simulink model "MS_QD2_QBPlat_R2021a"  (R2021a)
settings: Solver=ode2  StartTime=0.0  StopTime=inf  FixedStep=0.001  RelTol=1e-3  EnableMultiTasking=on
undefined symbols (not defined in the file): Host, localhost, qc_get_step_size
libraries: quarc_library x71, simulink x10, simulink_extras x2
(part 2 of 2)

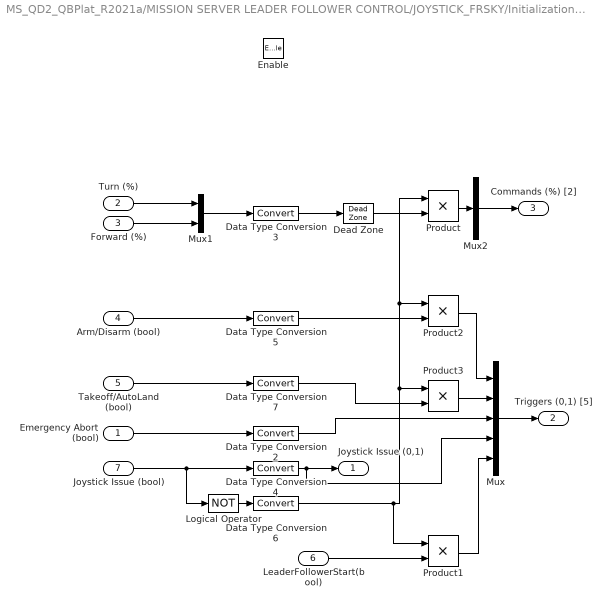
== system MS_QD2_QBPlat_R2021a/MISSION SERVER LEADER FOLLOWER CONTROL/JOYSTICK_FRSKY/Initialization and Conditioning ==
  Emergency Abort (bool) : Inport
  Turn (%) : Inport  Port=2
  Forward (%) : Inport  Port=3
  Arm/Disarm (bool) : Inport  Port=4
  Takeoff/AutoLand (bool) : Inport  Port=5
  LeaderFollowerStart(bool) : Inport  Port=6
  Joystick Issue (bool) : Inport  Port=7
  Enable : EnablePort  StatesWhenEnabling=reset
  Data Type Conversion{2..7} (6 alike) : DataTypeConversion
  Dead Zone : DeadZone  LowerValue=-0.01  UpperValue=0.01  SaturateOnIntegerOverflow=on
  Logical Operator : Logic  Operator=NOT  AllPortsSameDT=off  OutDataTypeStr=boolean
  Mux : Mux  Inputs=5
  Mux1 : Mux  Inputs=2
  Mux2 : Mux  Inputs=1
  Product{,1..3} (4 alike) : Product
  Joystick Issue (0,1) : Outport  InitialOutput=0  VectorParamsAs1DForOutWhenUnconnected=off
  Triggers (0,1) [5] : Outport  Port=2  InitialOutput=0  VectorParamsAs1DForOutWhenUnconnected=off
  Commands (%) [2] : Outport  Port=3  InitialOutput=0  VectorParamsAs1DForOutWhenUnconnected=off
  wires:
  Joystick Issue (bool)/1 -> Data Type Conversion4/1, Logical Operator/1
  Mux1/1 -> Data Type Conversion3/1
  Turn (%)/1 -> Mux1/1
  Forward (%)/1 -> Mux1/2
  Data Type Conversion4/1 -> Joystick Issue (0,1)/1, Mux/4
  Emergency Abort (bool)/1 -> Data Type Conversion2/1
  Data Type Conversion3/1 -> Dead Zone/1
  Arm/Disarm (bool)/1 -> Data Type Conversion5/1
  Mux/1 -> Triggers (0,1) [5]/1
  Data Type Conversion2/1 -> Mux/3
  Logical Operator/1 -> Data Type Conversion6/1
  Product/1 -> Mux2/1
  Dead Zone/1 -> Product/2
  Data Type Conversion6/1 -> Product3/1, Product2/1, Product/1, Product1/1
  Product2/1 -> Mux/1
  Data Type Conversion5/1 -> Product2/2
  Takeoff/AutoLand (bool)/1 -> Data Type Conversion7/1
  Product3/1 -> Mux/2
  Data Type Conversion7/1 -> Product3/2
  Mux2/1 -> Commands (%) [2]/1
  LeaderFollowerStart(bool)/1 -> Product1/2
  Product1/1 -> Mux/5

== system MS_QD2_QBPlat_R2021a/MISSION SERVER LEADER FOLLOWER CONTROL/JOYSTICK_FRSKY/Pulse Check ==
  note: For this subsystem we will count the number of new pulses. The data can be considered enabled once the count of new signals has gone beyond 2. This will enable the Initializing and conditioning subsystem.
  new : Inport
  Compare : quarc_library/Logic Operations/Compare  operator=>=  output_data_type=boolean
      settings: SourceProductName=QUARC Targets
  Pulse Check : Constant
  "pulse count " : Subsystem  TreatAsAtomicUnit=on
  signal enable : Outport  InitialOutput=0  VectorParamsAs1DForOutWhenUnconnected=off
  wires:
  Compare/1 -> signal enable/1
  Pulse Check/1 -> Compare/2
  new/1 -> "pulse count "/Trigger
  "pulse count "/1(Number of Pulses) -> Compare/1

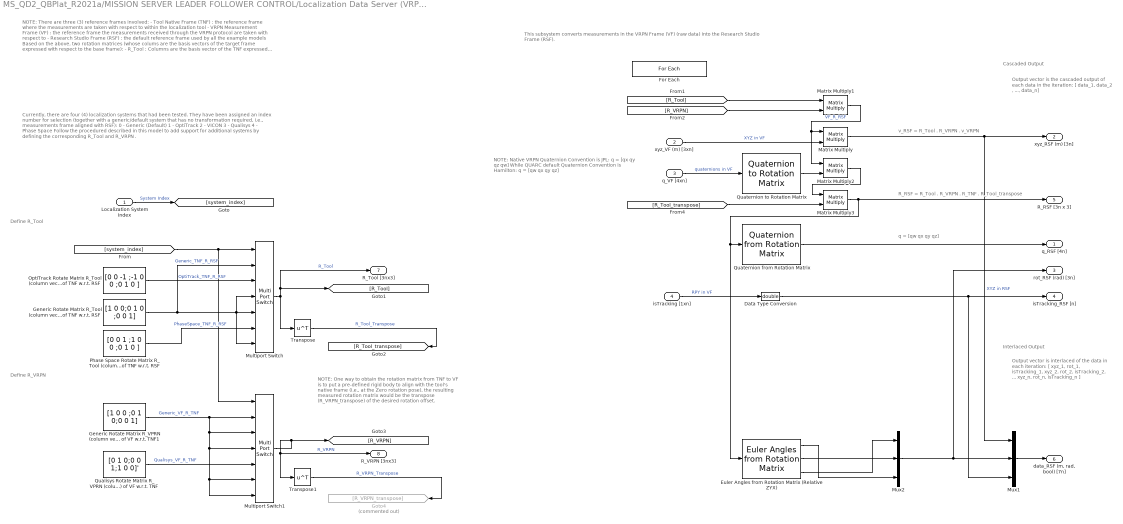
== system MS_QD2_QBPlat_R2021a/MISSION SERVER LEADER FOLLOWER CONTROL/Localization Data Server (VRPN) /For Each Subsystem (Convention Correction: Motive Frame to Research Studio Frame)1 ==
  note: R_RSF = R_Tool . R_VRPN . R_TNF . R_Tool_transpose
  note: v_RSF = R_Tool . R_VRPN . v_VRPN
  note: Define R_VRPN
  note: Currently, there are four (4) localization systems that had been tested. They have been assigned an index number for selection (together with a generic/default system that has no transformation required, i.e., measurements frame aligned with RSF):
      |
      | 0 - Generic (Default)
      | 1 - OptiTrack
      | 2 - VICON
      | 3 - Qualisys
      | 4 - Phase Space
      |
      | Follow the procedured described in this model to add support for additional systems by defining the corresponding R_Tool and R_VRPN .
  note: Define R_Tool
  note: NOTE:
      | There are three (3) reference frames involved:
      |
      | - Tool Native Frame (TNF) : the reference frame where the measurements are taken with respect to within the localization tool
      | - VRPN Measurement Frame (VF) : the reference frame the measurements received through the VRPN protocol are taken with respect to
      | - Research Studio Frame (RSF) : the default reference frame used by all the example models
      |
      | Based on the above, two rotation matrices (whose colums are the basis vectors of the target frame expressed with respect to the base frame):
      |
      | - R_Tool : Columns are the basis vector of the TNF expressed with respect to the RSF
      | - R_VPRN : Columns are the basis vector of the VRPN frame with respect to the TNF
      |
      | If all of the reference are aligned, then both R_Tool and R_VRPN will be a 3x3 identity matrices.
  note: NOTE:
      | One way to obtain the rotation matrix from TNF to VF
      | is to put a pre-defined rigid body to align with the tool's
      | native frame (i.e., at the Zero rotation pose), the resulting
      | measured rotation matrix would be the transpose (R_VRPN_transpose) of the desired rotation
      | offset.
  note: NOTE: Native VRPN Quaternion Convention is JPL:
      | q = [qx qy qz qw]
      |
      | While QUARC default Quaternion Convention is Hamilton:
      | q = [qw qx qy qz]
  note: Output vector is interlaced of the data
      | in each iteration:
      |
      | [ xyz_1, rot_1, isTracking_1,
      |   xyz_2, rot_2, isTracking_2,
      |   ...
      |   xyz_n, rot_n, isTracking_n ]
  note: Interlaced Output
  note: Output vector is the cascaded output of
      | each data in the iteration:
      | [ data_1, data_2 , ..., data_n]
  note: Cascaded Output
  note: q = [qw qx qy qz]
  note: This subsystem converts measurements in the VRPN Frame (VF) (raw data) into the Research Studio Frame (RSF).
  Localization System Index : Inport
  xyz_VF (m) [3xn] : Inport  Port=2  Partition=on  PartitionDimension=2  PartitionWidth=1  PartitionOffset=0
  q_VF [4xn] : Inport  Port=3  Partition=on  PartitionDimension=2  PartitionWidth=1  PartitionOffset=0
  isTracking [1xn] : Inport  Port=4  Partition=on  PartitionDimension=2  PartitionWidth=1  PartitionOffset=0
  " Generic Rotate Matrix R_VPRN (column vectors are basis vectors) of VF w.r.t. TNF1" : Constant  Value=[1 0 0 ;0 1 0;0 0 1]  VectorParams1D=off
  " Qualisys Rotate Matrix R_VPRN (column vectors are basis vectors) of VF w.r.t. TNF" : Constant  Value=[0 1 0;0 0 1;1 0 0]'  VectorParams1D=off
  Data Type Conversion : DataTypeConversion  OutDataTypeStr=double
  Euler Angles from Rotation Matrix (Relative ZYX) : quarc_library/Math Operations/Matrices/Euler Angles from Rotation Matrix  menu_order=Relative Z-Y-X
      settings: SourceProductName=QUARC Targets
  For Each : ForEach  DisableCoverage=on
  Generic Rotate Matrix R_Tool (column vectors are basis vectors) of TNF w.r.t. RSF : Constant  Value=[1 0 0;0 1 0 ;0 0 1]  VectorParams1D=off
  Goto4 : Goto  Commented=on  GotoTag=R_VRPN_transpose
  Matrix Multiply{,1..3} (4 alike) : Product  Multiplication=Matrix(*)
  Multiport Switch : MultiPortSwitch  DataPortOrder=Zero-based contiguous  Inputs=5  DataPortForDefault=Additional data port  DiagnosticForDefault=None  zeroidx=on
  Multiport Switch1 : MultiPortSwitch  DataPortOrder=Zero-based contiguous  Inputs=5  DataPortForDefault=Additional data port  DiagnosticForDefault=None  zeroidx=on
  Mux1 : Mux  Inputs=3
  Mux2 : Mux  Inputs=3
  OptiTrack Rotate Matrix R_Tool (column vectors are basis vectors) of TNF w.r.t. RSF : Constant  Value=[0 0 -1 ;-1 0 0 ;0 1 0 ]  VectorParams1D=off
  Phase Space Rotate Matrix R_Tool (column vectors are basis vectors) of TNF w.r.t. RSF : Constant  Value=[0 0 1 ;1 0 0 ;0 1 0 ]  VectorParams1D=off
  Quaternion from Rotation Matrix : quarc_library/Math Operations/Quaternions/Quaternion from Rotation Matrix
      settings: SourceProductName=QUARC Targets
  Quaternion to Rotation Matrix : quarc_library/Math Operations/Quaternions/Quaternion to Rotation Matrix
      settings: SourceProductName=QUARC Targets
  Transpose : Math  Operator=transpose  SaturateOnIntegerOverflow=on
  Transpose1 : Math  Operator=transpose  SaturateOnIntegerOverflow=on
  q_RSF [4n] : Outport  ConcatenationDimension=1
  xyz_RSF (m) [3n] : Outport  Port=2  ConcatenationDimension=1
  rot_RSF (rad) [3n] : Outport  Port=3  ConcatenationDimension=1
  isTracking_RSF [n] : Outport  Port=4  ConcatenationDimension=1
  R_RSF [3n x 3] : Outport  Port=5  ConcatenationDimension=1
  "data_RSF (m, rad, bool) [7n]" : Outport  Port=6  ConcatenationDimension=1
  R_Tool [3nx3] : Outport  Port=7  ConcatenationDimension=1
  R_VRPN [3nx3] : Outport  Port=8  ConcatenationDimension=1
  wires:
  q_VF [4xn]/1 -> Quaternion to Rotation Matrix/1  "quaternions in VF"
  Matrix Multiply/1 -> xyz_RSF (m) [3n]/1, Mux1/1  "XYZ in RSF"
  xyz_VF (m) [3xn]/1 -> Matrix Multiply/2  "XYZ in VF"
  isTracking [1xn]/1 -> Data Type Conversion/1  "RPY in VF"
  Mux1/1 -> "data_RSF (m, rad, bool) [7n]"/1
  Data Type Conversion/1 -> Mux1/3, isTracking_RSF [n]/1
  Euler Angles from Rotation Matrix (Relative ZYX)/3 -> Mux2/1
  Euler Angles from Rotation Matrix (Relative ZYX)/1 -> Mux2/3
  Euler Angles from Rotation Matrix (Relative ZYX)/2 -> Mux2/2
  Mux2/1 -> Mux1/2, rot_RSF (rad) [3n]/1
  Quaternion to Rotation Matrix/1 -> Matrix Multiply2/2
  Matrix Multiply2/1 -> Matrix Multiply3/1
  Quaternion from Rotation Matrix/1 -> q_RSF [4n]/1
  Generic Rotate Matrix R_Tool (column vectors are basis vectors) of TNF w.r.t. RSF/1 -> Multiport Switch/4, Multiport Switch/5, Multiport Switch/7, Multiport Switch/2  "Generic_TNF_R_RSF"
  OptiTrack Rotate Matrix R_Tool (column vectors are basis vectors) of TNF w.r.t. RSF/1 -> Multiport Switch/3  "OptiTrack_TNF_R_RSF"
  " Generic Rotate Matrix R_VPRN (column vectors are basis vectors) of VF w.r.t. TNF1"/1 -> Multiport Switch1/6, Multiport Switch1/7, Multiport Switch1/4, Multiport Switch1/3, Multiport Switch1/2  "Generic_VF_R_TNF"
  " Qualisys Rotate Matrix R_VPRN (column vectors are basis vectors) of VF w.r.t. TNF"/1 -> Multiport Switch1/5  "Qualisys_VF_R_TNF"
  [system_index] -> Multiport Switch1/1, Multiport Switch/1
  Multiport Switch/1 -> R_Tool [3nx3]/1, [R_Tool], Transpose/1  "R_Tool"
  Transpose/1 -> [R_Tool_transpose]  "R_Tool_Transpose"
  Multiport Switch1/1 -> R_VRPN [3nx3]/1, Transpose1/1, [R_VRPN]  "R_VRPN"
  Transpose1/1 -> Goto4/1  "R_VRPN_Transpose"
  [R_Tool] -> Matrix Multiply1/1
  [R_VRPN] -> Matrix Multiply1/2
  Matrix Multiply1/1 -> Matrix Multiply2/1, Matrix Multiply/1  "VF_R_RSF"
  [R_Tool_transpose] -> Matrix Multiply3/2
  Matrix Multiply3/1 -> Euler Angles from Rotation Matrix (Relative ZYX)/1, Quaternion from Rotation Matrix/1, R_RSF [3n x 3]/1
  Localization System Index/1 -> [system_index]  "System Index"
  Phase Space Rotate Matrix R_Tool (column vectors are basis vectors) of TNF w.r.t. RSF/1 -> Multiport Switch/6  "PhaseSpace_TNF_R_RSF"

== system MS_QD2_QBPlat_R2021a/MISSION SERVER LEADER FOLLOWER CONTROL/StopAllSignal/Subsystem ==
  Signal : Inport
  Delay : Delay  DelayLength=4
  Stop with Message : quarc_library/Sinks/Error Handling/Stop with Message  message_type=Fixed error message  message_icon=Error  message=QDrone Stopped, Stop all Models
  Threshold : quarc_library/Discontinuities/Threshold  operator=>=  param_src=Specify via dialog  threshold=0.5  duration=1
      settings: SourceProductName=QUARC Targets
  Threshold1 : quarc_library/Discontinuities/Threshold  operator=>=  param_src=Specify via dialog  threshold=0.5  duration=.3
      settings: SourceProductName=QUARC Targets
  Triggered Subsystem1 : Subsystem  TreatAsAtomicUnit=on
  Triggered Subsystem2 : Subsystem  TreatAsAtomicUnit=on
  Stop : Outport
  wires:
  Triggered Subsystem2/1(StopAllModels) -> Stop/1
  Signal/1 -> Threshold1/1, Threshold/1
  Threshold1/1 -> Triggered Subsystem2/Trigger
  Threshold/1 -> Triggered Subsystem1/Trigger, Delay/1
  Delay/1 -> Stop with Message/1

== system MS_QD2_QBPlat_R2021a/MISSION SERVER LEADER FOLLOWER CONTROL/StopAllSignal/Subsystem1 ==
  Signal : Inport
  Delay : Delay  DelayLength=4
  Stop with Message : quarc_library/Sinks/Error Handling/Stop with Message  message_type=Fixed error message  message_icon=Error  message=Joystick triggers not back
  Threshold : quarc_library/Discontinuities/Threshold  operator=>=  param_src=Specify via dialog  threshold=0.5  duration=3
      settings: SourceProductName=QUARC Targets
  Threshold1 : quarc_library/Discontinuities/Threshold  operator=>=  param_src=Specify via dialog  threshold=0.5  duration=2
      settings: SourceProductName=QUARC Targets
  Triggered Subsystem1 : Subsystem  TreatAsAtomicUnit=on
  Triggered Subsystem2 : Subsystem  TreatAsAtomicUnit=on
  Stop : Outport
  wires:
  Triggered Subsystem2/1(StopAllModels) -> Stop/1
  Signal/1 -> Threshold1/1, Threshold/1
  Threshold1/1 -> Triggered Subsystem2/Trigger
  Threshold/1 -> Triggered Subsystem1/Trigger, Delay/1
  Delay/1 -> Stop with Message/1

== system MS_QD2_QBPlat_R2021a/MISSION SERVER LEADER FOLLOWER CONTROL/StopAllSignal/Subsystem2 ==
  Signal : Inport
  Delay : Delay  DelayLength=4
  Stop with Message : quarc_library/Sinks/Error Handling/Stop with Message  message_type=Fixed error message  message_icon=Error  message=Not Tracking on start
  Threshold : quarc_library/Discontinuities/Threshold  operator=>=  param_src=Specify via dialog  threshold=0.5  duration=4
      settings: SourceProductName=QUARC Targets
  Threshold1 : quarc_library/Discontinuities/Threshold  operator=>=  param_src=Specify via dialog  threshold=0.5  duration=3
      settings: SourceProductName=QUARC Targets
  Triggered Subsystem1 : Subsystem  TreatAsAtomicUnit=on
  Triggered Subsystem2 : Subsystem  TreatAsAtomicUnit=on
  Stop : Outport
  wires:
  Triggered Subsystem2/1(StopAllModels) -> Stop/1
  Signal/1 -> Threshold1/1, Threshold/1
  Threshold1/1 -> Triggered Subsystem2/Trigger
  Threshold/1 -> Triggered Subsystem1/Trigger, Delay/1
  Delay/1 -> Stop with Message/1

== system MS_QD2_QBPlat_R2021a/MISSION SERVER LEADER FOLLOWER CONTROL/StopAllSignal/Subsystem3 ==
  Signal : Inport
  Delay : Delay  DelayLength=4
  Stop with Message : quarc_library/Sinks/Error Handling/Stop with Message  message_type=Fixed error message  message_icon=Error  message=Emergency stop triggered
  Threshold : quarc_library/Discontinuities/Threshold  operator=>=  param_src=Specify via dialog  threshold=0.5  duration=2
      settings: SourceProductName=QUARC Targets
  Threshold1 : quarc_library/Discontinuities/Threshold  operator=>=  param_src=Specify via dialog  threshold=0.5  duration=.5
      settings: SourceProductName=QUARC Targets
  Triggered Subsystem1 : Subsystem  TreatAsAtomicUnit=on
  Triggered Subsystem2 : Subsystem  TreatAsAtomicUnit=on
  Stop : Outport
  wires:
  Triggered Subsystem2/1(StopAllModels) -> Stop/1
  Signal/1 -> Threshold1/1, Threshold/1
  Threshold1/1 -> Triggered Subsystem2/Trigger
  Threshold/1 -> Triggered Subsystem1/Trigger, Delay/1
  Delay/1 -> Stop with Message/1

== system MS_QD2_QBPlat_R2021a/MISSION SERVER LEADER FOLLOWER CONTROL/StopAllSignal/Subsystem4 ==
  note: FrSky Issue Fix
  Signal : Inport
  Compare To Constant : simulink/Logic and Bit Operations/Compare To Constant  relop=>=  const=1  OutDataTypeStr=boolean
  Delay : Delay  DelayLength=4
  Product : Product
  Stop with Message : quarc_library/Sinks/Error Handling/Stop with Message  message_type=Fixed error message  message_icon=Error  message=Autoland Triggered
  Threshold : quarc_library/Discontinuities/Threshold  operator=>=  param_src=Specify via dialog  threshold=0.5  duration=1
      settings: SourceProductName=QUARC Targets
  Threshold1 : quarc_library/Discontinuities/Threshold  operator=>=  param_src=Specify via dialog  threshold=0.5  duration=.3
      settings: SourceProductName=QUARC Targets
  Threshold2 : quarc_library/Discontinuities/Threshold  operator=>=  param_src=Specify via dialog  threshold=0.5  duration=10
      settings: SourceProductName=QUARC Targets
  Time : quarc_library/Sources/Time/Time  time_source=Wall clock  sample_time=qc_get_step_size
  Triggered Subsystem1 : Subsystem  TreatAsAtomicUnit=on
  Triggered Subsystem2 : Subsystem  TreatAsAtomicUnit=on
  Triggered Subsystem3 : Subsystem  TreatAsAtomicUnit=on
  Stop : Outport
  wires:
  Triggered Subsystem2/1(StopAllModels) -> Stop/1
  Threshold2/1 -> Threshold1/1, Threshold/1
  Threshold1/1 -> Triggered Subsystem2/Trigger
  Threshold/1 -> Triggered Subsystem1/Trigger, Delay/1
  Triggered Subsystem3/1(Autoland Triggered) -> Threshold2/1
  Delay/1 -> Stop with Message/1
  Compare To Constant/1 -> Product/1
  Signal/1 -> Product/2
  Time/1 -> Compare To Constant/1
  Product/1 -> Triggered Subsystem3/Trigger

== system MS_QD2_QBPlat_R2021a/MISSION SERVER LEADER FOLLOWER CONTROL/StopAllSignal/Subsystem5 ==
  Signal : Inport
  Delay : Delay  DelayLength=4
  Stop with Message : quarc_library/Sinks/Error Handling/Stop with Message  message_type=Fixed error message  message_icon=Error  message=Robots not looking towards the wall
  Threshold : quarc_library/Discontinuities/Threshold  operator=>=  param_src=Specify via dialog  threshold=0.5  duration=2
      settings: SourceProductName=QUARC Targets
  Threshold1 : quarc_library/Discontinuities/Threshold  operator=>=  param_src=Specify via dialog  threshold=0.5  duration=1
      settings: SourceProductName=QUARC Targets
  Triggered Subsystem1 : Subsystem  TreatAsAtomicUnit=on
  Triggered Subsystem2 : Subsystem  TreatAsAtomicUnit=on
  Stop : Outport
  wires:
  Triggered Subsystem2/1(StopAllModels) -> Stop/1
  Signal/1 -> Threshold1/1, Threshold/1
  Threshold1/1 -> Triggered Subsystem2/Trigger
  Threshold/1 -> Triggered Subsystem1/Trigger, Delay/1
  Delay/1 -> Stop with Message/1

== system MS_QD2_QBPlat_R2021a/MISSION SERVER LEADER FOLLOWER CONTROL/Subsystem5/Triggered Subsystem1 ==
  Time (s) : Inport
  Trigger : TriggerPort  VariantControl=(inherit)
  Print2 : quarc_library/User Interface/Standard I//O/Print  format_string=[ %lf ] (s): DRONE ARMED \n  max_code_units=512  optimization=Minimizing latency  sample_time=-1  active=off
      settings: SourceProductName=QUARC Targets
  Terminator : Terminator
  Terminator1 : Terminator
  wires:
  Print2/2 -> Terminator/1
  Print2/1 -> Terminator1/1
  Time (s)/1 -> Print2/1

== system MS_QD2_QBPlat_R2021a/MISSION SERVER LEADER FOLLOWER CONTROL/Subsystem5/Triggered Subsystem2 ==
  Time (s) : Inport
  Trigger : TriggerPort  VariantControl=(inherit)
  Print2 : quarc_library/User Interface/Standard I//O/Print  format_string=[ %lf ] (s): DRONE TAKEOFF \n  max_code_units=512  optimization=Minimizing latency  sample_time=-1  active=off
      settings: SourceProductName=QUARC Targets
  Terminator : Terminator
  Terminator1 : Terminator
  wires:
  Time (s)/1 -> Print2/1
  Print2/1 -> Terminator1/1
  Print2/2 -> Terminator/1

== system MS_QD2_QBPlat_R2021a/MISSION SERVER LEADER FOLLOWER CONTROL/Subsystem5/Triggered Subsystem3 ==
  Time (s) : Inport
  Trigger : TriggerPort  VariantControl=(inherit)
  Print2 : quarc_library/User Interface/Standard I//O/Print  format_string=[ %lf ] (s): EMERGENCY STOP TRIGGERED \n  max_code_units=512  optimization=Minimizing latency  sample_time=-1  active=off
      settings: SourceProductName=QUARC Targets
  Terminator : Terminator
  Terminator1 : Terminator
  wires:
  Time (s)/1 -> Print2/1
  Print2/1 -> Terminator1/1
  Print2/2 -> Terminator/1

== system MS_QD2_QBPlat_R2021a/MISSION SERVER LEADER FOLLOWER CONTROL/Subsystem5/Triggered Subsystem4 ==
  Time (s) : Inport
  Trigger : TriggerPort  VariantControl=(inherit)
  Print2 : quarc_library/User Interface/Standard I//O/Print  format_string=[ %lf ] (s): JOYSTICK ISSUE \n  max_code_units=512  optimization=Minimizing latency  sample_time=-1  active=off
      settings: SourceProductName=QUARC Targets
  Terminator : Terminator
  Terminator1 : Terminator
  wires:
  Print2/1 -> Terminator1/1
  Print2/2 -> Terminator/1
  Time (s)/1 -> Print2/1

== system MS_QD2_QBPlat_R2021a/MISSION SERVER LEADER FOLLOWER CONTROL/Subsystem5/Triggered Subsystem5 ==
  Time (s) : Inport
  Trigger : TriggerPort  VariantControl=(inherit)
  Print2 : quarc_library/User Interface/Standard I//O/Print  format_string=[ %lf ] (s): START FOLLOWING \n  max_code_units=512  optimization=Minimizing latency  sample_time=-1  active=off
      settings: SourceProductName=QUARC Targets
  Terminator : Terminator
  Terminator1 : Terminator
  wires:
  Time (s)/1 -> Print2/1
  Print2/2 -> Terminator/1
  Print2/1 -> Terminator1/1

== system MS_QD2_QBPlat_R2021a/MISSION SERVER LEADER FOLLOWER CONTROL/Subsystem5/Triggered Subsystem6 ==
  Time (s) : Inport
  Trigger : TriggerPort  TriggerType=falling  VariantControl=(inherit)
  Print2 : quarc_library/User Interface/Standard I//O/Print  format_string=[ %lf ] (s): STOP FOLLOWING \n  max_code_units=512  optimization=Minimizing latency  sample_time=-1  active=off
      settings: SourceProductName=QUARC Targets
  Terminator : Terminator
  Terminator1 : Terminator
  wires:
  Time (s)/1 -> Print2/1
  Print2/2 -> Terminator/1
  Print2/1 -> Terminator1/1

== system MS_QD2_QBPlat_R2021a/MISSION SERVER LEADER FOLLOWER CONTROL/Subsystem5/Triggered Subsystem7 ==
  Time (s) : Inport
  Trigger : TriggerPort  TriggerType=falling  VariantControl=(inherit)
  Print2 : quarc_library/User Interface/Standard I//O/Print  format_string=[ %lf ] (s): DRONE LANDING \n  max_code_units=512  optimization=Minimizing latency  sample_time=-1  active=off
      settings: SourceProductName=QUARC Targets
  Terminator : Terminator
  Terminator1 : Terminator
  wires:
  Time (s)/1 -> Print2/1
  Print2/1 -> Terminator1/1
  Print2/2 -> Terminator/1

== system MS_QD2_QBPlat_R2021a/MISSION SERVER LEADER FOLLOWER CONTROL/JOYSTICK_FRSKY/Pulse Check/pulse count  ==
  Trigger : TriggerPort  VariantControl=Variant
  Constant1 : Constant  Value=0
  Increment Stored Integer : simulink/Additional Math & Discrete/Additional Math: Increment - Decrement/Increment Stored Integer
  Sum : Sum  Inputs=|++
  Unit Delay : UnitDelay  SampleTime=-1  HasFrameUpgradeWarning=on
  Number of Pulses : Outport  VectorParamsAs1DForOutWhenUnconnected=off
  wires:
  Constant1/1 -> Sum/1
  Sum/1 -> Increment Stored Integer/1
  Unit Delay/1 -> Sum/2
  Increment Stored Integer/1 -> Unit Delay/1, Number of Pulses/1

== system MS_QD2_QBPlat_R2021a/MISSION SERVER LEADER FOLLOWER CONTROL/StopAllSignal/Subsystem/Triggered Subsystem1 ==
  Trigger : TriggerPort  VariantControl=(inherit)
  Print : quarc_library/User Interface/Standard I//O/Print  format_string="Communication with QDrone Stopped, stopping all models  \\n"  max_code_units=512  optimization=Minimizing latency  sample_time=-1  active=off
      settings: SourceProductName=QUARC Targets

== system MS_QD2_QBPlat_R2021a/MISSION SERVER LEADER FOLLOWER CONTROL/StopAllSignal/Subsystem/Triggered Subsystem2 ==
  Trigger : TriggerPort  VariantControl=(inherit)
  Constant : Constant
  StopAllModels : Outport  InitialOutput=[0]
  wires:
  Constant/1 -> StopAllModels/1

== system MS_QD2_QBPlat_R2021a/MISSION SERVER LEADER FOLLOWER CONTROL/StopAllSignal/Subsystem1/Triggered Subsystem1 ==
  Trigger : TriggerPort  VariantControl=(inherit)
  Print : quarc_library/User Interface/Standard I//O/Print  format_string="Joystick triggers not back - Place them away from you and run again  \\n"  max_code_units=512  optimization=Minimizing latency  sample_time=-1  active=off
      settings: SourceProductName=QUARC Targets

== system MS_QD2_QBPlat_R2021a/MISSION SERVER LEADER FOLLOWER CONTROL/StopAllSignal/Subsystem1/Triggered Subsystem2 ==
  Trigger : TriggerPort  VariantControl=(inherit)
  Constant : Constant
  StopAllModels : Outport  InitialOutput=[0]
  wires:
  Constant/1 -> StopAllModels/1

== system MS_QD2_QBPlat_R2021a/MISSION SERVER LEADER FOLLOWER CONTROL/StopAllSignal/Subsystem2/Triggered Subsystem1 ==
  Trigger : TriggerPort  VariantControl=(inherit)
  Print : quarc_library/User Interface/Standard I//O/Print  format_string="Not tracking on start - Make sure correct vehicles are used  \\n"  max_code_units=512  optimization=Minimizing latency  sample_time=-1  active=off
      settings: SourceProductName=QUARC Targets

== system MS_QD2_QBPlat_R2021a/MISSION SERVER LEADER FOLLOWER CONTROL/StopAllSignal/Subsystem2/Triggered Subsystem2 ==
  Trigger : TriggerPort  VariantControl=(inherit)
  Constant : Constant
  StopAllModels : Outport  InitialOutput=[0]
  wires:
  Constant/1 -> StopAllModels/1

== system MS_QD2_QBPlat_R2021a/MISSION SERVER LEADER FOLLOWER CONTROL/StopAllSignal/Subsystem3/Triggered Subsystem1 ==
  Trigger : TriggerPort  VariantControl=(inherit)
  Print : quarc_library/User Interface/Standard I//O/Print  format_string="Emergency stop pressed  \\n"  max_code_units=512  optimization=Minimizing latency  sample_time=-1  active=off
      settings: SourceProductName=QUARC Targets

== system MS_QD2_QBPlat_R2021a/MISSION SERVER LEADER FOLLOWER CONTROL/StopAllSignal/Subsystem3/Triggered Subsystem2 ==
  Trigger : TriggerPort  VariantControl=(inherit)
  Constant : Constant
  StopAllModels : Outport  InitialOutput=[0]
  wires:
  Constant/1 -> StopAllModels/1

== system MS_QD2_QBPlat_R2021a/MISSION SERVER LEADER FOLLOWER CONTROL/StopAllSignal/Subsystem4/Triggered Subsystem1 ==
  Trigger : TriggerPort  VariantControl=(inherit)
  Print : quarc_library/User Interface/Standard I//O/Print  format_string="Stopped due to drone landing  \\n"  max_code_units=512  optimization=Minimizing latency  sample_time=-1  active=off
      settings: SourceProductName=QUARC Targets

== system MS_QD2_QBPlat_R2021a/MISSION SERVER LEADER FOLLOWER CONTROL/StopAllSignal/Subsystem4/Triggered Subsystem2 ==
  Trigger : TriggerPort  VariantControl=(inherit)
  Constant : Constant
  StopAllModels : Outport  InitialOutput=[0]
  wires:
  Constant/1 -> StopAllModels/1

== system MS_QD2_QBPlat_R2021a/MISSION SERVER LEADER FOLLOWER CONTROL/StopAllSignal/Subsystem4/Triggered Subsystem3 ==
  Trigger : TriggerPort  TriggerType=falling  VariantControl=(inherit)
  Constant : Constant
  Autoland Triggered : Outport  InitialOutput=[0]
  wires:
  Constant/1 -> Autoland Triggered/1

== system MS_QD2_QBPlat_R2021a/MISSION SERVER LEADER FOLLOWER CONTROL/StopAllSignal/Subsystem5/Triggered Subsystem1 ==
  Trigger : TriggerPort  VariantControl=(inherit)
  Print : quarc_library/User Interface/Standard I//O/Print  format_string=One of the vehicles not placed correctly. Camera should look at back wall. \n  max_code_units=512  optimization=Minimizing latency  sample_time=-1  active=off
      settings: SourceProductName=QUARC Targets

== system MS_QD2_QBPlat_R2021a/MISSION SERVER LEADER FOLLOWER CONTROL/StopAllSignal/Subsystem5/Triggered Subsystem2 ==
  Trigger : TriggerPort  VariantControl=(inherit)
  Constant : Constant
  StopAllModels : Outport  InitialOutput=[0]
  wires:
  Constant/1 -> StopAllModels/1

== matlab function MS_QD2_QBPlat_R2021a/MISSION SERVER LEADER FOLLOWER CONTROL/QBotData/Extract Object Data ==
  data: data input; position output; orientation output; index input; tracking output
function [position, orientation, tracking] = fcn(data, index)

n = length(data)/7;

if (index<=0)||(index>n)
    position = zeros(1,3); orientation = zeros(1,3); tracking = 0;
else
    position = [data(index*7 -6) data(index*7 -5) data(index*7 -4)];
    orientation = [data(index*7 -3) data(index*7 -2) data(index*7 -1)];
    tracking = data(index*7);
end

== matlab function MS_QD2_QBPlat_R2021a/MISSION SERVER LEADER FOLLOWER CONTROL/QDroneData/Extract Object Data ==
  data: data input; position output; orientation output; index input; tracking output

function [position, orientation, tracking] = fcn(data, index)

n = length(data)/7;


% position = data((index-1)*3 + 1: (index-1)*3 + 3);
% orientation = data( 3*n + 3*(index-1) + 1: 3*n + 3*(index-1) + 3);
% tracking = data(end-n+index - 1);


if (index<=0)||(index>n)
    position = zeros(1,3); orientation = zeros(1,3); tracking = 0;
else
    position = [data(index*7 -6) data(index*7 -5) data(index*7 -4)];
    orientation = [data(index*7 -3) data(index*7 -2) data(index*7 -1)];
    tracking = data(index*7);
end

== matlab function MS_QD2_QBPlat_R2021a/Communication/Detect Communication loss/MATLAB Function ==
  data: time input; stream_connection_loss output; state input; error input
function stream_connection_loss  = fcn(time, state, error)

stream_connection_loss = 0;
if time > 1
    if ~((state == 2)&&(error >= 0))
        % stream connection is not established correctly
        stream_connection_loss = 1;
    end
end
